simulink model "PreChargeChart"  (R2023b)
settings: Solver=VariableStepAuto  StartTime=0.0  StopTime=1  RelTol=1e-3
settings Model: Creator=romul  LastModifiedBy=OWNER
settings DebuggingCC: UnderSpecifiedDimensionMsg=warning

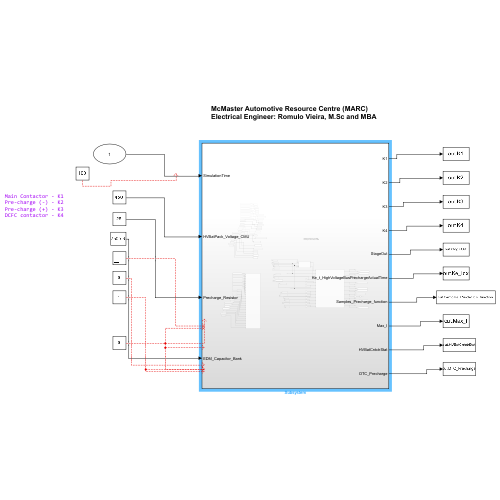
[thumbnail: Simulink's stored preview of the top-level diagram]
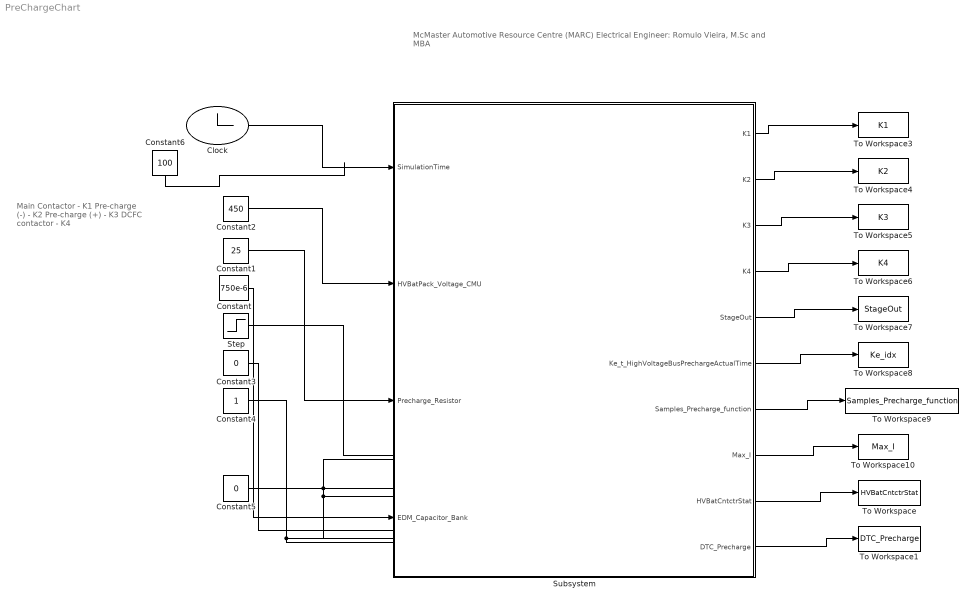
== system PreChargeChart ==
  note: McMaster Automotive Resource Centre (MARC)
      | Electrical Engineer: Romulo Vieira, M.Sc and MBA
  note: Main Contactor - K1
      | Pre-charge (-) - K2
      | Pre-charge (+) - K3
      | DCFC contactor - K4
  Clock : Clock
  Constant : Constant  Value=750e-6
  Constant1 : Constant  Value=25
  Constant2 : Constant  Value=450
  Constant3 : Constant  Value=0
  Constant4 : Constant
  Constant5 : Constant  Value=0
  Constant6 : Constant  Value=100
  Step : Step  Time=0.5  SampleTime=0.001
  Subsystem : Subsystem  SystemSampleTime=0.001
  To Workspace : ToWorkspace  VariableName=HVBatCntctrStat  SaveFormat=Timeseries  SampleTime=-1
  To Workspace1 : ToWorkspace  VariableName=DTC_Precharge  SaveFormat=Timeseries  SampleTime=-1
  To Workspace10 : ToWorkspace  VariableName=Max_I  SampleTime=-1
  To Workspace3 : ToWorkspace  VariableName=K1  SampleTime=-1
  To Workspace4 : ToWorkspace  VariableName=K2  SampleTime=-1
  To Workspace5 : ToWorkspace  VariableName=K3  SampleTime=-1
  To Workspace6 : ToWorkspace  VariableName=K4  SampleTime=-1
  To Workspace7 : ToWorkspace  VariableName=StageOut  SampleTime=-1
  To Workspace8 : ToWorkspace  VariableName=Ke_idx  SampleTime=-1
  To Workspace9 : ToWorkspace  VariableName=Samples_Precharge_function  SampleTime=-1
  wires:
  Constant6/1 -> ?
  Subsystem/6(Ke_t_HighVoltageBusPrechargeActualTime) -> To Workspace8/1
  Constant4/1 -> ?
  Subsystem/5(StageOut) -> To Workspace7/1
  Constant3/1 -> ?
  Subsystem/4(K4) -> To Workspace6/1
  Step/1 -> ?
  Clock/1 -> Subsystem/1(SimulationTime)
  Constant1/1 -> Subsystem/3(Precharge_Resistor)
  Subsystem/3(K3) -> To Workspace5/1
  Constant2/1 -> Subsystem/2(HVBatPack_Voltage_CMU)
  Constant/1 -> Subsystem/4(EDM_Capacitor_Bank)
  Constant5/1 -> ?
  Subsystem/10(DTC_Precharge) -> To Workspace1/1
  Subsystem/2(K2) -> To Workspace4/1
  Subsystem/1(K1) -> To Workspace3/1
  Subsystem/7(Samples_Precharge_function) -> To Workspace9/1
  Subsystem/8(Max_I) -> To Workspace10/1
  Subsystem/9(HVBatCntctrStat) -> To Workspace/1

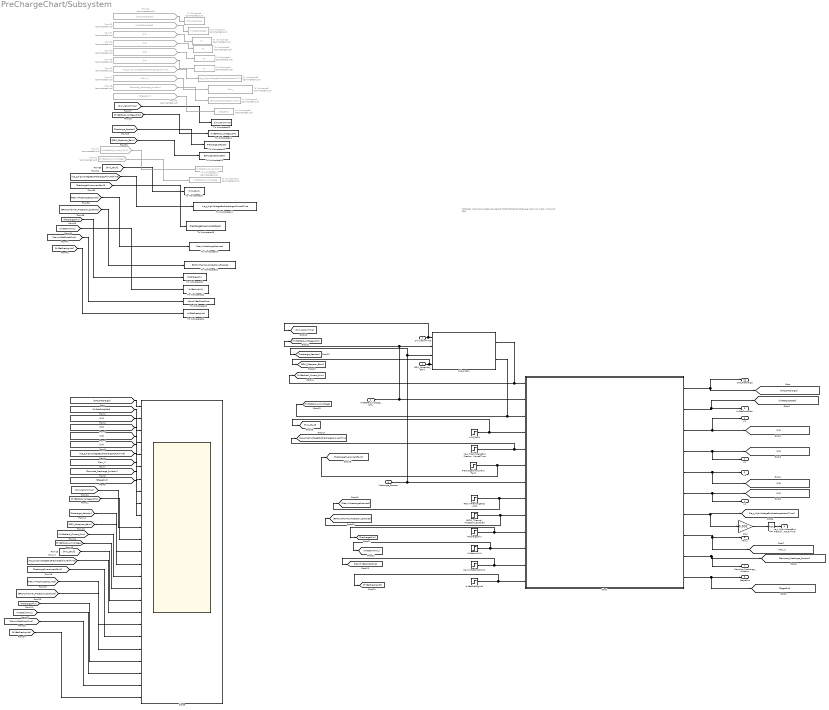
== system PreChargeChart/Subsystem ==
  note: McMaster Automotive Resource Centre (MARC)
      | Electrical Engineer: Romulo Vieira, M.Sc and MBA
  SimulationTime : Inport
  HVBatPack_Voltage_CMU : Inport  Port=2
  Precharge_Resistor : Inport  Port=3
  EDM_Capacitor_Bank : Inport  Port=4
  BPCM_Thermal_Protection_Enabled : Step  Time=550  SampleTime=0.001
  Chart : Stateflow chart  TreatAsAtomicUnit=on
  From25 : From  Commented=on  GotoTag=DTC_Precharge
  From26 : From  Commented=on  GotoTag=HVBatCntctrStat
  From31 : From  Commented=on  GotoTag=HVBatPack_Current_Prim
  From32 : From  Commented=on  GotoTag=HVBatPack_LinkVoltage
  From37 : From  Commented=on  GotoTag=K1
  From43 : From  Commented=on  GotoTag=K2
  From44 : From  Commented=on  GotoTag=K3
  From45 : From  Commented=on  GotoTag=K4
  From46 : From  Commented=on  GotoTag=Ke_t_HighVoltageBusPrechargeActualTime
  From47 : From  Commented=on  GotoTag=Max_I
  From48 : From  Commented=on  GotoTag=Samples_Precharge_function
  From49 : From  Commented=on  GotoTag=StageOut
  Gain : Gain  Gain=0.001
  HVBatInitHVIL : Step  Before=1  SampleTime=0
  HVBatPrechgInbt : Step  After=0  SampleTime=0
  HVIL_Fault : Step  After=0  SampleTime=0
  Ke_t_HighVoltageBusPrechargeAllowedTime : Step  Before=100  After=100  SampleTime=0
  MainHVBatCntctrCmd : Step  Time=500  SampleTime=0.001
  Max : MinMax  Function=max
  PrechargeAllw : Step  Time=0.4  SampleTime=0.001
  PrechargeOvercurrentFault : Step  After=0  SampleTime=0
  RetryInPrechargeOccurred : Step  After=0  SampleTime=0
  Scope : Scope  NumInputPorts=25
  Subsystem : Subsystem
  To Workspace : ToWorkspace  Commented=on  VariableName=DTC_Precharge  SaveFormat=Timeseries  SampleTime=-1
  To Workspace1 : ToWorkspace  Commented=on  VariableName=HVBatCntctrStat  SaveFormat=Timeseries  SampleTime=-1
  To Workspace10 : ToWorkspace  VariableName=SimulationTime  SaveFormat=Timeseries  SampleTime=-1
  To Workspace11 : ToWorkspace  VariableName=HVBatPack_Voltage_CMU  SaveFormat=Timeseries  SampleTime=-1
  To Workspace12 : ToWorkspace  VariableName=Precharge_Resistor  SaveFormat=Timeseries  SampleTime=-1
  To Workspace13 : ToWorkspace  VariableName=EDM_Capacitor_Bank  SaveFormat=Timeseries  SampleTime=-1
  To Workspace14 : ToWorkspace  Commented=on  VariableName=HVBatPack_Current_Prim  SaveFormat=Timeseries  SampleTime=-1
  To Workspace15 : ToWorkspace  Commented=on  VariableName=HVBatPack_LinkVoltage  SaveFormat=Timeseries  SampleTime=-1
  To Workspace16 : ToWorkspace  VariableName=HVIL_Fault  SaveFormat=Timeseries  SampleTime=-1
  To Workspace17 : ToWorkspace  VariableName=Ke_t_HighVoltageBusPrechargeAllowedTime  SaveFormat=Timeseries  SampleTime=-1
  To Workspace18 : ToWorkspace  VariableName=PrechargeOvercurrentFault  SaveFormat=Timeseries  SampleTime=-1
  To Workspace19 : ToWorkspace  VariableName=RetryInPrechargeOccurred  SaveFormat=Timeseries  SampleTime=-1
  To Workspace2 : ToWorkspace  Commented=on  VariableName=K1  SaveFormat=Timeseries  SampleTime=-1
  To Workspace20 : ToWorkspace  VariableName=BPCM_Thermal_Protection_Enabled  SaveFormat=Timeseries  SampleTime=-1
  To Workspace21 : ToWorkspace  VariableName=PrechargeAllw  SaveFormat=Timeseries  SampleTime=-1
  To Workspace22 : ToWorkspace  VariableName=HVBatInitHVIL  SaveFormat=Timeseries  SampleTime=-1
  To Workspace23 : ToWorkspace  VariableName=MainHVBatCntctrCmd  SaveFormat=Timeseries  SampleTime=-1
  To Workspace24 : ToWorkspace  VariableName=HVBatPrechgInbt  SaveFormat=Timeseries  SampleTime=-1
  To Workspace3 : ToWorkspace  Commented=on  VariableName=K2  SaveFormat=Timeseries  SampleTime=-1
  To Workspace4 : ToWorkspace  Commented=on  VariableName=K3  SaveFormat=Timeseries  SampleTime=-1
  To Workspace5 : ToWorkspace  Commented=on  VariableName=K4  SaveFormat=Timeseries  SampleTime=-1
  To Workspace6 : ToWorkspace  Commented=on  VariableName=Ke_t_HighVoltageBusPrechargeActualTime  SaveFormat=Timeseries  SampleTime=-1
  To Workspace7 : ToWorkspace  Commented=on  VariableName=Max_I  SaveFormat=Timeseries  SampleTime=-1
  To Workspace8 : ToWorkspace  Commented=on  VariableName=Samples_Precharge_function  SaveFormat=Timeseries  SampleTime=-1
  To Workspace9 : ToWorkspace  Commented=on  VariableName=StageOut  SaveFormat=Timeseries  SampleTime=-1
  K1 : Outport
  K2 : Outport  Port=2
  K3 : Outport  Port=3
  K4 : Outport  Port=4
  StageOut : Outport  Port=5
  Ke_t_HighVoltageBusPrechargeActualTime : Outport  Port=6
  Samples_Precharge_function : Outport  Port=7
  Max_I : Outport  Port=8
  HVBatCntctrStat : Outport  Port=9
  DTC_Precharge : Outport  Port=10
  wires:
  RetryInPrechargeOccurred/1 -> [RetryInPrechargeOccurred], Chart/8(RetryInPrechargeOccurred)
  HVIL_Fault/1 -> [HVIL_Fault], Chart/4(HVIL_Fault)
  HVBatPrechgInbt/1 -> [HVBatPrechgInbt], Chart/13(HVBatPrechgInbt)
  Subsystem/2(HVBatPack_LinkVoltage) -> Chart/3(HVBatPack_LinkVoltage), [HVBatPack_LinkVoltage]
  Chart/5(K3) -> [K3], K3/1
  Chart/9(Samples_Precharge_function) -> [Samples_Precharge_function], Samples_Precharge_function/1
  HVBatInitHVIL/1 -> [HVBatInitHVIL], Chart/11(HVBatInitHVIL)
  SimulationTime/1 -> [SimulationTime], Subsystem/1(SimulationTime)
  EDM_Capacitor_Bank/1 -> [EDM_Capacitor_Bank], Subsystem/4(EDM_Capacitor_Bank)
  HVBatPack_Voltage_CMU/1 -> Subsystem/2(HVBatPack_Voltage_CMU), [HVBatPack_Voltage_CMU], Chart/2(HVBatPack_Voltage_CMU)
  Precharge_Resistor/1 -> Chart/7(Precharge_Resistor), [Precharge_Resistor], Subsystem/3(Precharge_Resistor)
  Chart/2(HVBatCntctrStat) -> [HVBatCntctrStat], HVBatCntctrStat/1
  Subsystem/1(HVBatPack_Current_Prim) -> Chart/1(HVBatPack_Current_Prim), [HVBatPack_Current_Prim]
  Ke_t_HighVoltageBusPrechargeAllowedTime/1 -> [Ke_t_HighVoltageBusPrechargeAllowedTime], Chart/5(Ke_t_HighVoltageBusPrechargeAllowedTime)
  PrechargeOvercurrentFault/1 -> [PrechargeOvercurrentFault], Chart/6(PrechargeOvercurrentFault)
  PrechargeAllw/1 -> [PrechargeAllw], Chart/10(PrechargeAllw)
  Chart/8(Max_I) -> Max_I/1, [Max_I]
  BPCM_Thermal_Protection_Enabled/1 -> [BPCM_Thermal_Protection_Enabled], Chart/9(BPCM_Thermal_Protection_Enabled)
  MainHVBatCntctrCmd/1 -> [MainHVBatCntctrCmd], Chart/12(MainHVBatCntctrCmd)
  Chart/1(DTC_Precharge) -> DTC_Precharge/1, [DTC_Precharge]
  Chart/3(K1) -> K1/1, [K1]
  Chart/7(Ke_t_HighVoltageBusPrechargeActualTime) -> [Ke_t_HighVoltageBusPrechargeActualTime], Gain/1
  Chart/4(K2) -> [K2], K2/1
  Chart/6(K4) -> K4/1, [K4]
  Chart/10(StageOut) -> StageOut/1, [StageOut]
  Gain/1 -> Max/1
  Max/1 -> Ke_t_HighVoltageBusPrechargeActualTime/1
  [DTC_Precharge] -> Scope/1
  [HVBatCntctrStat] -> Scope/2
  [K1] -> Scope/3
  [K2] -> Scope/4
  [K3] -> Scope/5
  [K4] -> Scope/6
  [Ke_t_HighVoltageBusPrechargeActualTime] -> Scope/7
  [Max_I] -> Scope/8
  [Samples_Precharge_function] -> Scope/9
  [StageOut] -> Scope/10
  [SimulationTime] -> Scope/11
  [HVBatPack_Voltage_CMU] -> Scope/12
  [Precharge_Resistor] -> Scope/13
  [EDM_Capacitor_Bank] -> Scope/14
  [HVBatPack_Current_Prim] -> Scope/15
  [HVBatPack_LinkVoltage] -> Scope/16
  [HVIL_Fault] -> Scope/17
  [Ke_t_HighVoltageBusPrechargeAllowedTime] -> Scope/18
  [PrechargeOvercurrentFault] -> Scope/20
  [RetryInPrechargeOccurred] -> Scope/19
  [BPCM_Thermal_Protection_Enabled] -> Scope/21
  [PrechargeAllw] -> Scope/22
  [HVBatInitHVIL] -> Scope/23
  [MainHVBatCntctrCmd] -> Scope/24
  [HVBatPrechgInbt] -> Scope/25
  From46/1 -> To Workspace6/1
  [Precharge_Resistor] -> To Workspace12/1
  From26/1 -> To Workspace1/1
  [HVBatPrechgInbt] -> To Workspace24/1
  [MainHVBatCntctrCmd] -> To Workspace23/1
  [BPCM_Thermal_Protection_Enabled] -> To Workspace20/1
  [SimulationTime] -> To Workspace10/1
  [RetryInPrechargeOccurred] -> To Workspace19/1
  [Ke_t_HighVoltageBusPrechargeAllowedTime] -> To Workspace17/1
  [HVIL_Fault] -> To Workspace16/1
  [PrechargeAllw] -> To Workspace21/1
  From31/1 -> To Workspace14/1
  From49/1 -> To Workspace9/1
  [HVBatInitHVIL] -> To Workspace22/1
  [HVBatPack_Voltage_CMU] -> To Workspace11/1
  From37/1 -> To Workspace2/1
  From47/1 -> To Workspace7/1
  From32/1 -> To Workspace15/1
  [EDM_Capacitor_Bank] -> To Workspace13/1
  From48/1 -> To Workspace8/1
  From25/1 -> To Workspace/1
  From43/1 -> To Workspace3/1
  From44/1 -> To Workspace4/1
  [PrechargeOvercurrentFault] -> To Workspace18/1
  From45/1 -> To Workspace5/1

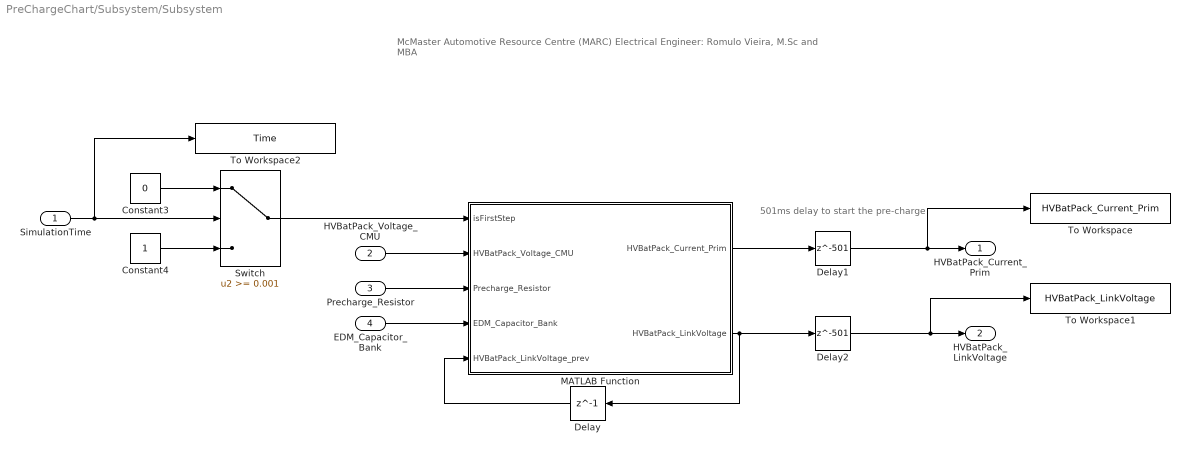
== system PreChargeChart/Subsystem/Subsystem ==
  note: 501ms delay to start the pre-charge
  note: McMaster Automotive Resource Centre (MARC)
      | Electrical Engineer: Romulo Vieira, M.Sc and MBA
  SimulationTime : Inport
  HVBatPack_Voltage_CMU : Inport  Port=2
  Precharge_Resistor : Inport  Port=3
  EDM_Capacitor_Bank : Inport  Port=4
  Constant3 : Constant  Value=0
  Constant4 : Constant
  Delay : Delay  DelayLength=1
  Delay1 : Delay  DelayLength=501
  Delay2 : Delay  DelayLength=501
  MATLAB Function : MATLAB Function  TreatAsAtomicUnit=on  SystemSampleTime=0.001
  Switch : Switch  Threshold=0.001  SaturateOnIntegerOverflow=off  InputSameDT=off
  To Workspace : ToWorkspace  VariableName=HVBatPack_Current_Prim  SampleTime=-1
  To Workspace1 : ToWorkspace  VariableName=HVBatPack_LinkVoltage  SampleTime=-1
  To Workspace2 : ToWorkspace  VariableName=Time  SampleTime=-1
  HVBatPack_Current_Prim : Outport
  HVBatPack_LinkVoltage : Outport  Port=2
  wires:
  MATLAB Function/1(HVBatPack_Current_Prim) -> Delay1/1
  Constant4/1 -> Switch/3
  EDM_Capacitor_Bank/1 -> MATLAB Function/4(EDM_Capacitor_Bank)
  Delay/1 -> MATLAB Function/5(HVBatPack_LinkVoltage_prev)
  Precharge_Resistor/1 -> MATLAB Function/3(Precharge_Resistor)
  Switch/1 -> MATLAB Function/1(isFirstStep)
  MATLAB Function/2(HVBatPack_LinkVoltage) -> Delay2/1, Delay/1
  HVBatPack_Voltage_CMU/1 -> MATLAB Function/2(HVBatPack_Voltage_CMU)
  Constant3/1 -> Switch/1
  SimulationTime/1 -> To Workspace2/1, Switch/2
  Delay1/1 -> To Workspace/1, HVBatPack_Current_Prim/1
  Delay2/1 -> To Workspace1/1, HVBatPack_LinkVoltage/1

== matlab function PreChargeChart/Subsystem/Subsystem/MATLAB Function ==
  data: isFirstStep input; HVBatPack_Current_Prim output; HVBatPack_Voltage_CMU input; HVBatPack_LinkVoltage output; Precharge_Resistor input; EDM_Capacitor_Bank input; HVBatPack_LinkVoltage_prev input
% McMaster Automotive Resource Centre (MARC)
% Electrical Engineer - Romulo Vieira, M.Sc and MBA, PhD Candidate
function [HVBatPack_Current_Prim, HVBatPack_LinkVoltage] = PreCharge(isFirstStep, HVBatPack_Voltage_CMU, Precharge_Resistor, EDM_Capacitor_Bank, HVBatPack_LinkVoltage_prev)
% PRECHARGESTEP - Compute pre-charge voltage and current for this time step
%
% Inputs:
%   Vpack         - Battery pack voltage (V)
%   Rprecharge    - Pre-charge resistor value (Ohms)
%   CdcLink       - DC link capacitance (F)
%   V_HVbus_prev  - Previous HV bus voltage (V)
%   isFirstStep   - Boolean flag (true at t=0, false otherwise)
%
% Outputs:
%   V_HVbus       - Updated HV bus voltage (V)
%   I_precharge   - Pre-charge current (A)

    dt = 0.001; % Sample time (s)
    tau = Precharge_Resistor * EDM_Capacitor_Bank;

    if isFirstStep == 1
        % On first step, force initial condition
        HVBatPack_LinkVoltage = 0;
        HVBatPack_Current_Prim = HVBatPack_Voltage_CMU / Precharge_Resistor;
    else
        % Normal RC discrete update
        HVBatPack_LinkVoltage = HVBatPack_Voltage_CMU - (HVBatPack_Voltage_CMU - HVBatPack_LinkVoltage_prev) * exp(-dt / tau);
        HVBatPack_Current_Prim = (HVBatPack_Voltage_CMU - HVBatPack_LinkVoltage) / Precharge_Resistor;
    end

end

== stateflow chart PreChargeChart/Subsystem/Chart ==
  state SignalNotAvailable
    entry:
    HVBatCntctrStat = 7;
    K1 = 0;
    K2 = 0;
    K3 = 0;
    K4 = 0;
    StageOut = 6;
    DTC_Precharge = 1;
  state Init
    entry:
    K1 = 0;
    K2 = 0;
    K3 = 0;
    K4 = 0;
    HVBatCntctrStat = 0;
    StageOut = 0;
    DTC_Precharge = 0;
    t_start = 0;
    t_counter = 0;
    idx = 1;
    fill_count = 0;
    stage2_count = 0;
    Ke_idx = -1;
    I_buffer = zeros(1, 100);
    V_buffer = zeros(1, 100);
    delta_samples = 0;
  state Precharge_Inhibited
    entry:
    K1 = 0;
    K2 = 0;
    K3 = 0;
    K4 = 0;
    HVBatCntctrStat = 4;
    DTC_Precharge = 1;
    StageOut = 5;
  state Precharging
    entry:
    K1 = 0;
    K2 = 1;
    K3 = 1;
    K4 = 0;
    HVBatCntctrStat = 1;
    StageOut = 1;
    during:
    V_buffer(idx) = HVBatPack_LinkVoltage;
    if fill_count == 0
    I_buffer(idx) = HVBatPack_Voltage_CMU / Rprecharge;
    else
    I_buffer(idx) = HVBatPack_Current_Prim;
    end
    idx = idx + 1;
    fill_count = fill_count + 1;
    if idx > 100
    idx = 1;
    end
    max_I = max(I_buffer);
    delta_samples = t_counter - t_start;
    if HVBatPack_LinkVoltage >= V_target && Ke_idx == -1
    Ke_idx = t_counter;
    end
  state Precharge_Failed
    entry:
    K1 = 0;
    K2 = 0;
    K3 = 0;
    K4 = 0;
    HVBatCntctrStat = 3;
    StageOut = 4;
  state Precharge_Mintime
    entry:
    K1 = 1;
    K2 = 1;
    K3 = 1;
    K4 = 0;
    HVBatCntctrStat = 1;
    StageOut = 2;
    stage2_count = 0;
    during:
    stage2_count = stage2_count + 1;
  state Closed
    entry:
    K1 = 1;
    K2 = 0;
    K3 = 0;
    K4 = 0;
    HVBatCntctrStat = 2;
    StageOut = 3;
    DTC_Precharge = 0;
    last_PrechargeAllw = PrechargeAllw;
  SignalNotAvailable -> Init : [MainHVBatCntctrCmd == 1 && HVBatInitHVIL == 1 && PrechargeAllw  == 1]{DTC_Precharge = 0;}
  (default) -> Init
  Init -> Precharge_Inhibited [order 1] : [BPCM_Thermal_Protection_Enabled == 1]
  Precharge_Inhibited -> Init : [BPCM_Thermal_Protection_Enabled == 0  && PrechargeAllw == 1]{DTC_Precharge = 0;}
  Closed -> Init : [MainHVBatCntctrCmd == 0 || (last_PrechargeAllw == 0 && PrechargeAllw == 1)]
  Precharge_Failed -> Init : [MainHVBatCntctrCmd == 0]
  Init -> Precharging [order 2] : [MainHVBatCntctrCmd == 1 && HVBatInitHVIL == 1 && PrechargeAllw == 1 && HVBatPrechgInbt == 0]{V_target = 0.95 * HVBatPack_Voltage_CMU; Rprecharge = Precharge_Resistor; t_start = t_counter;}
  Precharging -> Precharge_Failed [order 1] : [delta_samples > Ke_t_HighVoltageBusPrechargeAllowedTime || HVIL_Fault == 1 || PrechargeOvercurrentFault == 1 || RetryInPrechargeOccurred == 1]{DTC_Precharge = 1;}
  Precharging -> Precharge_Mintime [order 2] : [Ke_idx > 0 && delta_samples <= Ke_t_HighVoltageBusPrechargeAllowedTime && max_I > HVBatPack_Voltage_CMU / Rprecharge]{Ke_t_HighVoltageBusPrechargeActualTime = delta_samples; Max_I = max_I; Samples_Precharge_function = delta_samples;}
  Precharge_Mintime -> Closed : [stage2_count >= 5]
  data: HVBatPack_Current_Prim input; HVBatPack_Voltage_CMU input; HVBatPack_LinkVoltage input; HVIL_Fault input; Ke_t_HighVoltageBusPrechargeAllowedTime input; PrechargeOvercurrentFault input; Precharge_Resistor input; RetryInPrechargeOccurred input; DTC_Precharge output; HVBatCntctrStat output; K1 output; K2 output; K3 output; K4 output; Ke_t_HighVoltageBusPrechargeActualTime output; I_buffer local; idx local; t_start local; BPCM_Thermal_Protection_Enabled input; Max_I output; Samples_Precharge_function output; StageOut output; Ke_idx local; Rprecharge local; V_target local; delta_samples local; fill_count local; max_I local; stage2_count local; last_PrechargeAllw local; PrechargeAllw input; HVBatInitHVIL input; MainHVBatCntctrCmd input; HVBatPrechgInbt input; V_buffer local; t_counter local
